simulink model "Quadcopter_Modelling_SWETHA_RAVISELVAN"  (R2024b)
settings: Solver=FixedStepAuto  StartTime=0.0  StopTime=60  FixedStep=0.01  RelTol=1e-3
undefined symbols (not defined in the file): Ixx, Iyy, Izz, Kax, Kay, Kaz, l, m
settings Model: Creator=ros  LastModifiedBy=ros

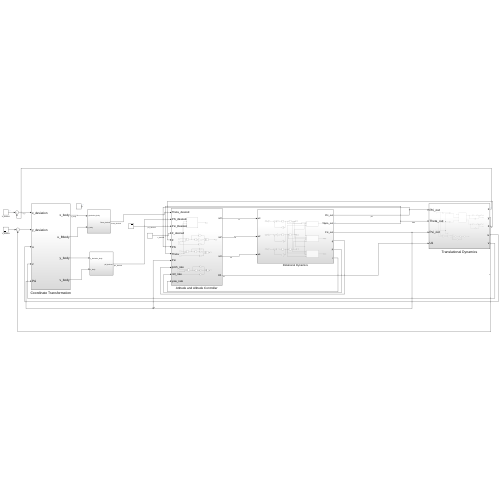
[thumbnail: Simulink's stored preview of the top-level diagram]
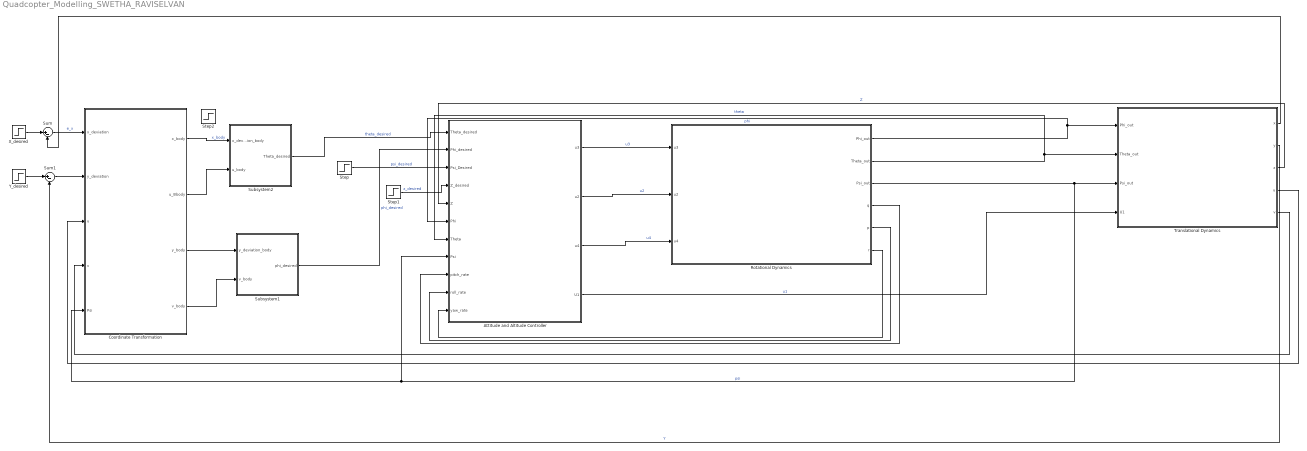
== system Quadcopter_Modelling_SWETHA_RAVISELVAN ==
  Attitude and Altitude Controller : Subsystem
  Coordinate Transformation : Subsystem
  Rotational Dynamics : Subsystem
  Step : Step  After=0  SampleTime=0
  Step1 : Step  After=-2  SampleTime=0
  Step2 : Step  After=0.3  SampleTime=0
  Subsystem1 : Subsystem
  Subsystem2 : Subsystem
  Sum : Sum  Inputs=|+-
  Sum1 : Sum  Inputs=|+-
  Translational Dynamics : Subsystem
  X_desired : Step  SampleTime=0
  Y_desired : Step  After=2  SampleTime=0
  wires:
  Coordinate Transformation/2(u_Bbody) -> Subsystem2/2(u_body)
  Rotational Dynamics/1(Phi_out) -> Translational Dynamics/1(Phi_out), Attitude and Altitude Controller/6(Phi)  "phi"
  Rotational Dynamics/2(Theta_out) -> Translational Dynamics/2(Theta_out), Attitude and Altitude Controller/7(Theta)  "theta"
  Rotational Dynamics/3(Psi_out) -> Attitude and Altitude Controller/8(Psi), Coordinate Transformation/5(Psi), Translational Dynamics/3(Psi_out)  "psi"
  Translational Dynamics/3(z) -> Attitude and Altitude Controller/5(Z)  "Z"
  X_desired/1 -> Sum/1
  Y_desired/1 -> Sum1/1
  Translational Dynamics/2(y) -> Sum1/2  "Y"
  Sum1/1 -> Coordinate Transformation/2(y_deviation)
  Sum/1 -> Coordinate Transformation/1(x_deviation)  "e_x"
  Coordinate Transformation/3(y_body) -> Subsystem1/1(y_deviation_body)
  Coordinate Transformation/4(v_body) -> Subsystem1/2(v_body)
  Rotational Dynamics/4(q) -> Attitude and Altitude Controller/9(pitch_rate)
  Rotational Dynamics/5(p) -> Attitude and Altitude Controller/10(roll_rate)
  Attitude and Altitude Controller/2(u2) -> Rotational Dynamics/2(u2)  "u2"
  Attitude and Altitude Controller/1(u3) -> Rotational Dynamics/1(u3)  "u3"
  Attitude and Altitude Controller/3(u4) -> Rotational Dynamics/3(u4)  "u4"
  Translational Dynamics/4(u) -> Coordinate Transformation/3(u)
  Translational Dynamics/5(v) -> Coordinate Transformation/4(v)
  Rotational Dynamics/6(r) -> Attitude and Altitude Controller/11(yaw_rate)
  Step/1 -> Attitude and Altitude Controller/3(Psi_Desired)  "psi_desired"
  Step1/1 -> Attitude and Altitude Controller/4(Z_desired)  "z_desired"
  Attitude and Altitude Controller/4(U1) -> Translational Dynamics/4(U1)  "u1"
  Subsystem1/1(phi_desired) -> Attitude and Altitude Controller/2(Phi_desired)  "phi_desired"
  Subsystem2/1(Theta_desired) -> Attitude and Altitude Controller/1(Theta_desired)  "theta_desired"
  Translational Dynamics/1(x) -> Sum/2
  Coordinate Transformation/1(x_body) -> Subsystem2/1(x_deviation_body)  "x_body"

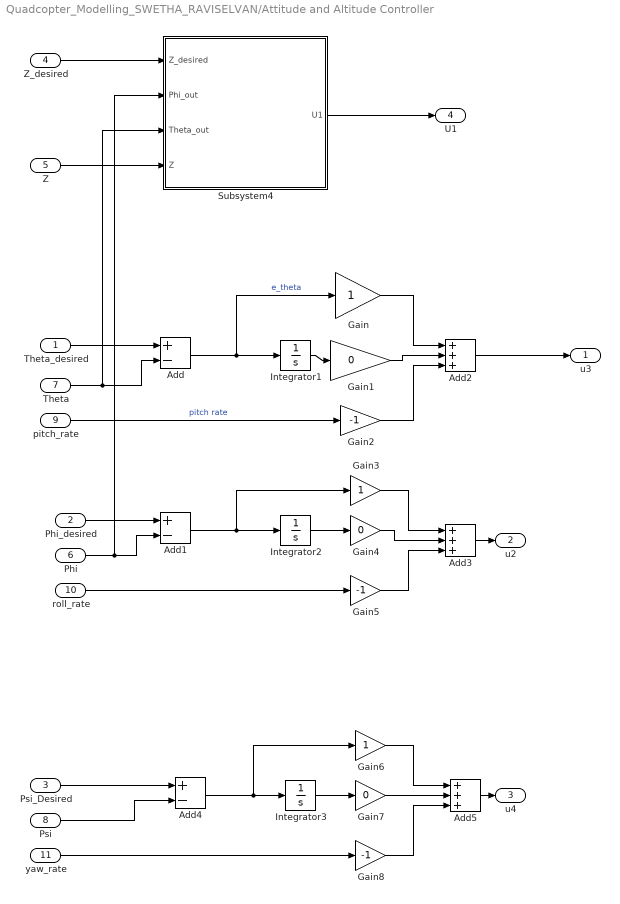
== system Quadcopter_Modelling_SWETHA_RAVISELVAN/Attitude and Altitude Controller ==
  Theta_desired : Inport
  Phi_desired : Inport  Port=2
  Psi_Desired : Inport  Port=3
  Z_desired : Inport  Port=4
  Z : Inport  Port=5
  Phi : Inport  Port=6
  Theta : Inport  Port=7
  Psi : Inport  Port=8
  pitch_rate : Inport  Port=9
  roll_rate : Inport  Port=10
  yaw_rate : Inport  Port=11
  Add : Sum  Inputs=+-
  Add1 : Sum  Inputs=+-
  Add2 : Sum  Inputs=+++
  Add3 : Sum  Inputs=+++
  Add4 : Sum  Inputs=+-
  Add5 : Sum  Inputs=+++
  Gain : Gain
  Gain1 : Gain  Gain=0
  Gain2 : Gain  Gain=-1
  Gain3 : Gain
  Gain4 : Gain  Gain=0
  Gain5 : Gain  Gain=-1
  Gain6 : Gain
  Gain7 : Gain  Gain=0
  Gain8 : Gain  Gain=-1
  Integrator1 : Integrator
  Integrator2 : Integrator
  Integrator3 : Integrator
  Subsystem4 : Subsystem
  u3 : Outport
  u2 : Outport  Port=2
  u4 : Outport  Port=3
  U1 : Outport  Port=4
  wires:
  pitch_rate/1 -> Gain2/1  "pitch rate"
  Integrator1/1 -> Gain1/1
  roll_rate/1 -> Gain5/1
  Gain3/1 -> Add3/1
  Gain8/1 -> Add5/3
  Gain5/1 -> Add3/3
  Add1/1 -> Gain3/1, Integrator2/1
  Add/1 -> Gain/1, Integrator1/1  "e_theta"
  Integrator3/1 -> Gain7/1
  Psi/1 -> Add4/2
  Psi_Desired/1 -> Add4/1
  Add2/1 -> u3/1
  Phi_desired/1 -> Add1/1
  Add3/1 -> u2/1
  Gain7/1 -> Add5/2
  Add4/1 -> Gain6/1, Integrator3/1
  yaw_rate/1 -> Gain8/1
  Gain6/1 -> Add5/1
  Add5/1 -> u4/1
  Integrator2/1 -> Gain4/1
  Gain4/1 -> Add3/2
  Subsystem4/1(U1) -> U1/1
  Z/1 -> Subsystem4/4(Z)
  Phi/1 -> Add1/2, Subsystem4/2(Phi_out)
  Theta/1 -> Add/2, Subsystem4/3(Theta_out)
  Gain/1 -> Add2/1
  Gain1/1 -> Add2/2
  Gain2/1 -> Add2/3
  Theta_desired/1 -> Add/1
  Z_desired/1 -> Subsystem4/1(Z_desired)

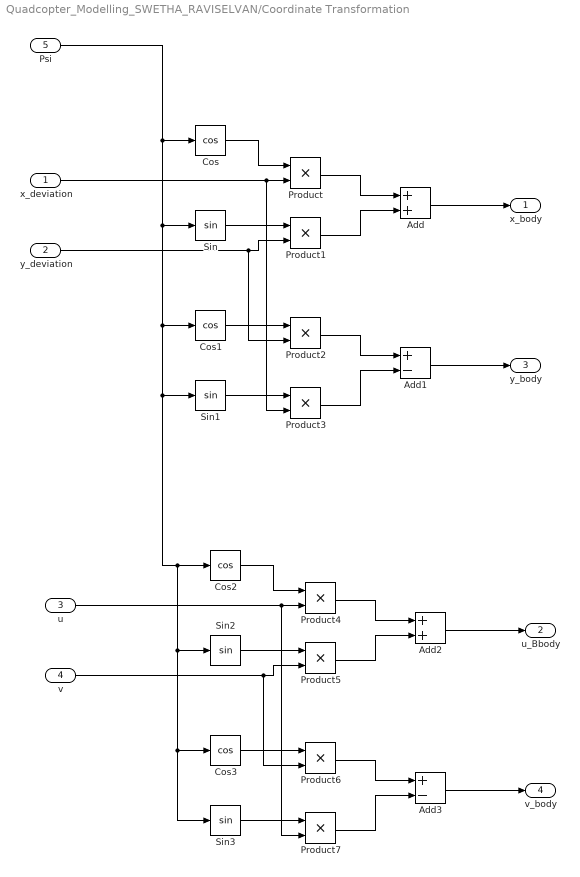
== system Quadcopter_Modelling_SWETHA_RAVISELVAN/Coordinate Transformation ==
  x_deviation : Inport
  y_deviation : Inport  Port=2
  u : Inport  Port=3
  v : Inport  Port=4
  Psi : Inport  Port=5
  Add : Sum
  Add1 : Sum  Inputs=+-
  Add2 : Sum
  Add3 : Sum  Inputs=+-
  Cos{,1..3} (4 alike) : Trigonometry  Operator=cos
  Product{,1..7} (8 alike) : Product
  Sin{,1..3} (4 alike) : Trigonometry
  x_body : Outport
  u_Bbody : Outport  Port=2
  y_body : Outport  Port=3
  v_body : Outport  Port=4
  wires:
  Sin1/1 -> Product3/1
  y_deviation/1 -> Product2/2, Product1/2
  x_deviation/1 -> Product3/2, Product/2
  Product1/1 -> Add/2
  Product3/1 -> Add1/2
  Cos/1 -> Product/1
  Sin/1 -> Product1/1
  Add1/1 -> y_body/1
  Product/1 -> Add/1
  Add/1 -> x_body/1
  Product2/1 -> Add1/1
  Cos1/1 -> Product2/1
  Cos3/1 -> Product6/1
  Product6/1 -> Add3/1
  Add2/1 -> u_Bbody/1
  Product4/1 -> Add2/1
  Add3/1 -> v_body/1
  Psi/1 -> Cos2/1, Sin2/1, Cos3/1, Sin3/1, Sin1/1, Cos1/1, Sin/1, Cos/1
  Sin2/1 -> Product5/1
  Cos2/1 -> Product4/1
  Product7/1 -> Add3/2
  Product5/1 -> Add2/2
  u/1 -> Product4/2, Product7/2
  v/1 -> Product5/2, Product6/2
  Sin3/1 -> Product7/1

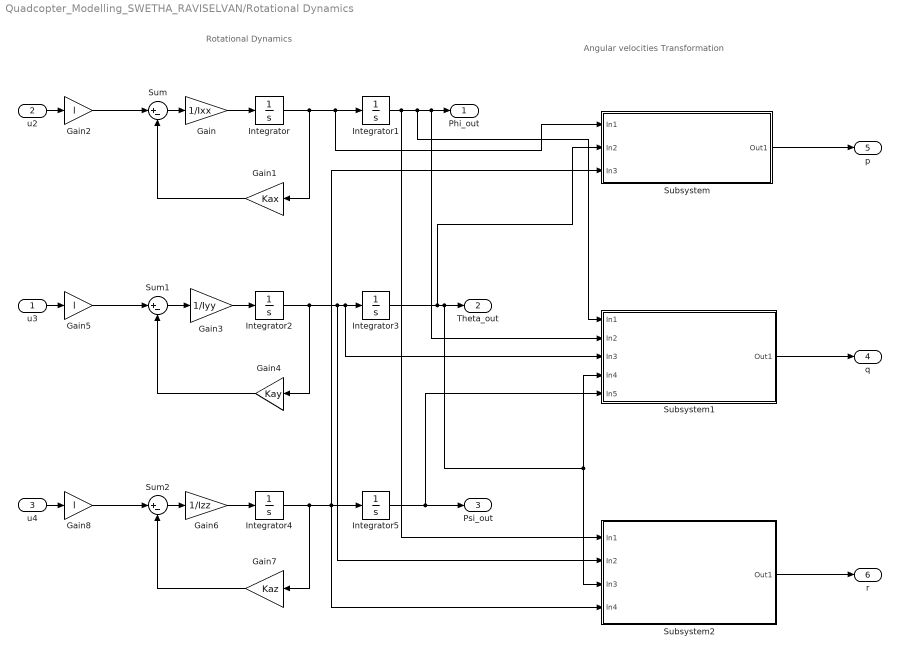
== system Quadcopter_Modelling_SWETHA_RAVISELVAN/Rotational Dynamics ==
  note: Rotational Dynamics
  note: Angular velocities Transformation
  u3 : Inport
  u2 : Inport  Port=2
  u4 : Inport  Port=3
  Gain : Gain  Gain=1/Ixx
  Gain1 : Gain  Gain=Kax
  Gain2 : Gain  Gain=l
  Gain3 : Gain  Gain=1/Iyy
  Gain4 : Gain  Gain=Kay
  Gain5 : Gain  Gain=l
  Gain6 : Gain  Gain=1/Izz
  Gain7 : Gain  Gain=Kaz
  Gain8 : Gain  Gain=l
  Integrator{,1..5} (6 alike) : Integrator
  Subsystem : Subsystem
  Subsystem1 : Subsystem
  Subsystem2 : Subsystem
  Sum : Sum  Inputs=|+-
  Sum1 : Sum  Inputs=|+-
  Sum2 : Sum  Inputs=|+-
  Phi_out : Outport
  Theta_out : Outport  Port=2
  Psi_out : Outport  Port=3
  q : Outport  Port=4
  p : Outport  Port=5
  r : Outport  Port=6
  wires:
  Gain7/1 -> Sum2/2
  Gain5/1 -> Sum1/1
  Gain4/1 -> Sum1/2
  Gain3/1 -> Integrator2/1
  Gain1/1 -> Sum/2
  Sum/1 -> Gain/1
  u4/1 -> Gain8/1
  Gain/1 -> Integrator/1
  u2/1 -> Gain2/1
  Sum1/1 -> Gain3/1
  Integrator5/1 -> Subsystem1/5(In5), Psi_out/1
  Gain8/1 -> Sum2/1
  Gain6/1 -> Integrator4/1
  u3/1 -> Gain5/1
  Sum2/1 -> Gain6/1
  Gain2/1 -> Sum/1
  Integrator/1 -> Gain1/1, Subsystem/1(In1), Integrator1/1
  Integrator2/1 -> Gain4/1, Subsystem2/2(In2), Subsystem1/3(In3), Integrator3/1
  Integrator1/1 -> Subsystem2/1(In1), Subsystem1/1(In1), Subsystem1/2(In2), Phi_out/1
  Integrator3/1 -> Subsystem/2(In2), Subsystem2/3(In3), Subsystem1/4(In4), Theta_out/1
  Integrator4/1 -> Gain7/1, Subsystem2/4(In4), Subsystem/3(In3), Integrator5/1
  Subsystem/1(Out1) -> p/1
  Subsystem1/1(Out1) -> q/1
  Subsystem2/1(Out1) -> r/1

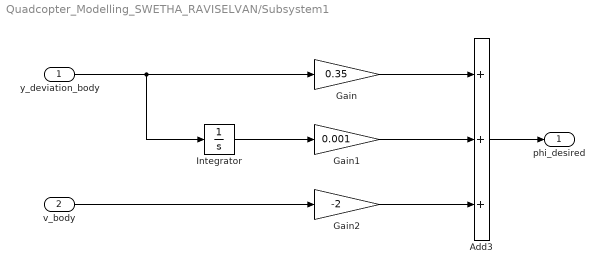
== system Quadcopter_Modelling_SWETHA_RAVISELVAN/Subsystem1 ==
  y_deviation_body : Inport
  v_body : Inport  Port=2
  Add3 : Sum  Inputs=+++
  Gain : Gain  Gain=0.35
  Gain1 : Gain  Gain=0.001
  Gain2 : Gain  Gain=-2
  Integrator : Integrator
  phi_desired : Outport
  wires:
  y_deviation_body/1 -> Gain/1, Integrator/1
  Gain/1 -> Add3/1
  Integrator/1 -> Gain1/1
  Gain1/1 -> Add3/2
  Add3/1 -> phi_desired/1
  v_body/1 -> Gain2/1
  Gain2/1 -> Add3/3

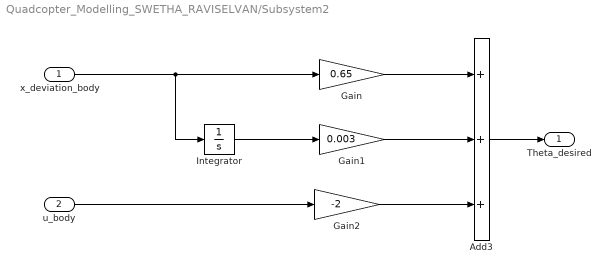
== system Quadcopter_Modelling_SWETHA_RAVISELVAN/Subsystem2 ==
  x_deviation_body : Inport
  u_body : Inport  Port=2
  Add3 : Sum  Inputs=+++
  Gain : Gain  Gain=0.65
  Gain1 : Gain  Gain=0.003
  Gain2 : Gain  Gain=-2
  Integrator : Integrator
  Theta_desired : Outport
  wires:
  u_body/1 -> Gain2/1
  Add3/1 -> Theta_desired/1
  Integrator/1 -> Gain1/1
  Gain/1 -> Add3/1
  x_deviation_body/1 -> Integrator/1, Gain/1
  Gain2/1 -> Add3/3
  Gain1/1 -> Add3/2

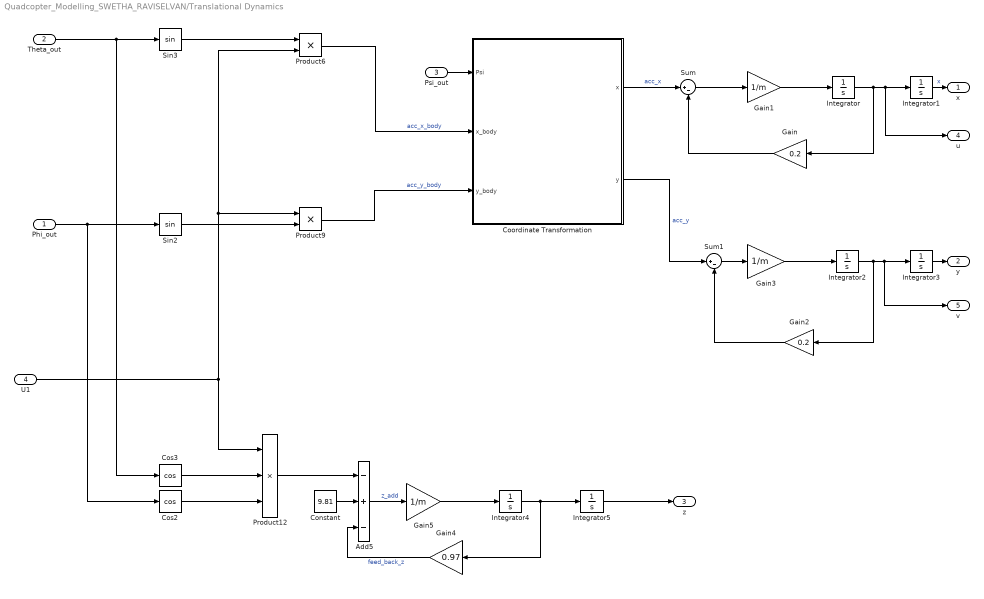
== system Quadcopter_Modelling_SWETHA_RAVISELVAN/Translational Dynamics ==
  Phi_out : Inport
  Theta_out : Inport  Port=2
  Psi_out : Inport  Port=3
  U1 : Inport  Port=4
  Add5 : Sum  Inputs=-+-
  Constant : Constant  Value=9.81
  Coordinate Transformation : Subsystem
  Cos2 : Trigonometry  Operator=cos
  Cos3 : Trigonometry  Operator=cos
  Gain : Gain  Gain=0.2
  Gain1 : Gain  Gain=1/m
  Gain2 : Gain  Gain=0.2
  Gain3 : Gain  Gain=1/m
  Gain4 : Gain  Gain=0.97
  Gain5 : Gain  Gain=1/m
  Integrator{,1..5} (6 alike) : Integrator
  Product12 : Product  Inputs=3
  Product6 : Product
  Product9 : Product
  Sin2 : Trigonometry
  Sin3 : Trigonometry
  Sum : Sum  Inputs=|+-
  Sum1 : Sum  Inputs=|+-
  x : Outport
  y : Outport  Port=2
  z : Outport  Port=3
  u : Outport  Port=4
  v : Outport  Port=5
  wires:
  Sin3/1 -> Product6/1
  Gain3/1 -> Integrator2/1
  Gain1/1 -> Integrator/1
  Integrator1/1 -> x/1  "x"
  Product12/1 -> Add5/1
  Theta_out/1 -> Cos3/1, Sin3/1
  Gain/1 -> Sum/2
  Integrator4/1 -> Gain4/1, Integrator5/1
  Constant/1 -> Add5/2
  Gain4/1 -> Add5/3  "feed_back_z"
  Sum/1 -> Gain1/1
  Gain5/1 -> Integrator4/1
  Integrator3/1 -> y/1
  Add5/1 -> Gain5/1  "z_add"
  Integrator5/1 -> z/1
  Sum1/1 -> Gain3/1
  Sin2/1 -> Product9/2
  Phi_out/1 -> Cos2/1, Sin2/1
  U1/1 -> Product6/2, Product9/1, Product12/1
  Psi_out/1 -> Coordinate Transformation/1(Psi)
  Gain2/1 -> Sum1/2
  Integrator/1 -> Gain/1, u/1, Integrator1/1
  Integrator2/1 -> v/1, Integrator3/1, Gain2/1
  Coordinate Transformation/1(x) -> Sum/1  "acc_x"
  Coordinate Transformation/2(y) -> Sum1/1  "acc_y"
  Product9/1 -> Coordinate Transformation/3(y_body)  "acc_y_body"
  Product6/1 -> Coordinate Transformation/2(x_body)  "acc_x_body"
  Cos3/1 -> Product12/2
  Cos2/1 -> Product12/3

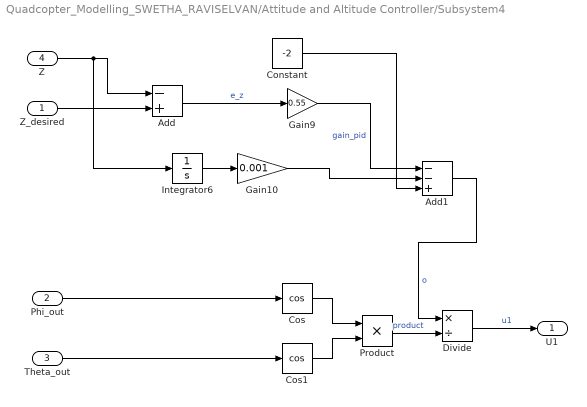
== system Quadcopter_Modelling_SWETHA_RAVISELVAN/Attitude and Altitude Controller/Subsystem4 ==
  Z_desired : Inport
  Phi_out : Inport  Port=2
  Theta_out : Inport  Port=3
  Z : Inport  Port=4
  Add : Sum  Inputs=-+
  Add1 : Sum  Inputs=--+
  Constant : Constant  Value=-2
  Cos : Trigonometry  Operator=cos
  Cos1 : Trigonometry  Operator=cos
  Divide : Product  Inputs=*/
  Gain10 : Gain  Gain=0.001
  Gain9 : Gain  Gain=0.55
  Integrator6 : Integrator
  Product : Product
  U1 : Outport
  wires:
  Phi_out/1 -> Cos/1
  Theta_out/1 -> Cos1/1
  Cos1/1 -> Product/2
  Add/1 -> Gain9/1  "e_z"
  Integrator6/1 -> Gain10/1
  Z/1 -> Integrator6/1, Add/1
  Cos/1 -> Product/1
  Z_desired/1 -> Add/2
  Product/1 -> Divide/2  "product"
  Add1/1 -> Divide/1  "o"
  Divide/1 -> U1/1  "u1"
  Gain10/1 -> Add1/2
  Gain9/1 -> Add1/1  "gain_pid"
  Constant/1 -> Add1/3

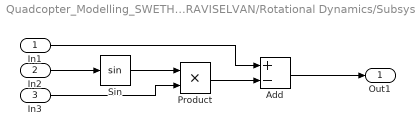
== system Quadcopter_Modelling_SWETHA_RAVISELVAN/Rotational Dynamics/Subsystem ==
  In1 : Inport
  In2 : Inport  Port=2
  In3 : Inport  Port=3
  Add : Sum  Inputs=+-
  Product : Product
  Sin : Trigonometry
  Out1 : Outport
  wires:
  Product/1 -> Add/2
  In1/1 -> Add/1
  Sin/1 -> Product/1
  In3/1 -> Product/2
  In2/1 -> Sin/1
  Add/1 -> Out1/1

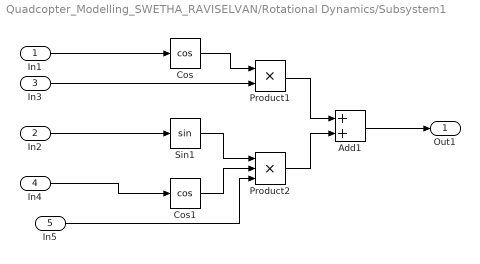
== system Quadcopter_Modelling_SWETHA_RAVISELVAN/Rotational Dynamics/Subsystem1 ==
  In1 : Inport
  In2 : Inport  Port=2
  In3 : Inport  Port=3
  In4 : Inport  Port=4
  In5 : Inport  Port=5
  Add1 : Sum
  Cos : Trigonometry  Operator=cos
  Cos1 : Trigonometry  Operator=cos
  Product1 : Product
  Product2 : Product  Inputs=3
  Sin1 : Trigonometry
  Out1 : Outport
  wires:
  In2/1 -> Sin1/1
  Product1/1 -> Add1/1
  Sin1/1 -> Product2/1
  In4/1 -> Cos1/1
  In3/1 -> Product1/2
  Cos/1 -> Product1/1
  Add1/1 -> Out1/1
  In5/1 -> Product2/3
  Cos1/1 -> Product2/2
  Product2/1 -> Add1/2
  In1/1 -> Cos/1

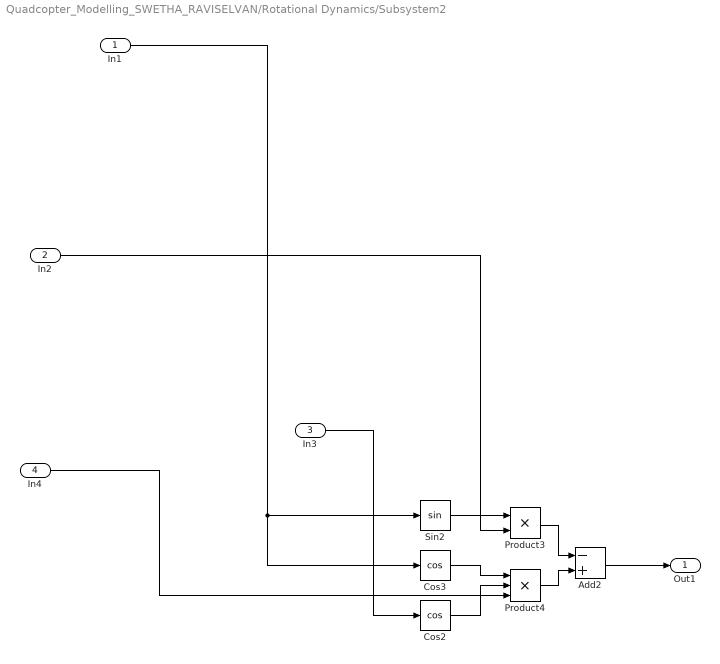
== system Quadcopter_Modelling_SWETHA_RAVISELVAN/Rotational Dynamics/Subsystem2 ==
  In1 : Inport
  In2 : Inport  Port=2
  In3 : Inport  Port=3
  In4 : Inport  Port=4
  Add2 : Sum  Inputs=-+
  Cos2 : Trigonometry  Operator=cos
  Cos3 : Trigonometry  Operator=cos
  Product3 : Product
  Product4 : Product  Inputs=3
  Sin2 : Trigonometry
  Out1 : Outport
  wires:
  Cos3/1 -> Product4/1
  In3/1 -> Cos2/1
  Product3/1 -> Add2/1
  In2/1 -> Product3/2
  Sin2/1 -> Product3/1
  Cos2/1 -> Product4/2
  Product4/1 -> Add2/2
  In4/1 -> Product4/3
  Add2/1 -> Out1/1
  In1/1 -> Cos3/1, Sin2/1

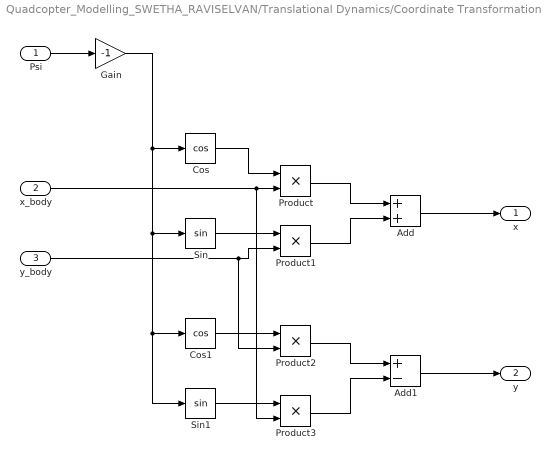
== system Quadcopter_Modelling_SWETHA_RAVISELVAN/Translational Dynamics/Coordinate Transformation ==
  Psi : Inport
  x_body : Inport  Port=2
  y_body : Inport  Port=3
  Add : Sum
  Add1 : Sum  Inputs=+-
  Cos : Trigonometry  Operator=cos
  Cos1 : Trigonometry  Operator=cos
  Gain : Gain  Gain=-1
  Product{,1..3} (4 alike) : Product
  Sin : Trigonometry
  Sin1 : Trigonometry
  x : Outport
  y : Outport  Port=2
  wires:
  Sin1/1 -> Product3/1
  y_body/1 -> Product2/2, Product1/2
  x_body/1 -> Product3/2, Product/2
  Product1/1 -> Add/2
  Product3/1 -> Add1/2
  Cos/1 -> Product/1
  Sin/1 -> Product1/1
  Add1/1 -> y/1
  Product/1 -> Add/1
  Add/1 -> x/1
  Product2/1 -> Add1/1
  Cos1/1 -> Product2/1
  Psi/1 -> Gain/1
  Gain/1 -> Sin1/1, Cos1/1, Sin/1, Cos/1
